simulink model "DSB_TC_Transmitter"  (R2022a)
settings: Solver=FixedStepDiscrete  StartTime=0.0  StopTime=inf  RelTol=1e-3
libraries: dspsnks4 x1, commanapbnd3 x1, dspvision x1, dspsigops x1, matrix_library x1
settings Model: Creator=vovan  LastModifiedBy=vovan

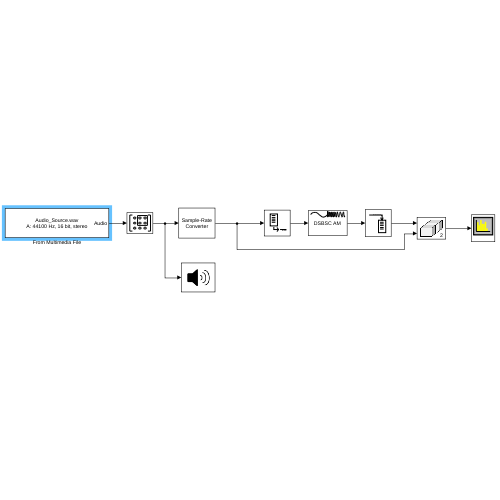
[thumbnail: Simulink's stored preview of the top-level diagram]
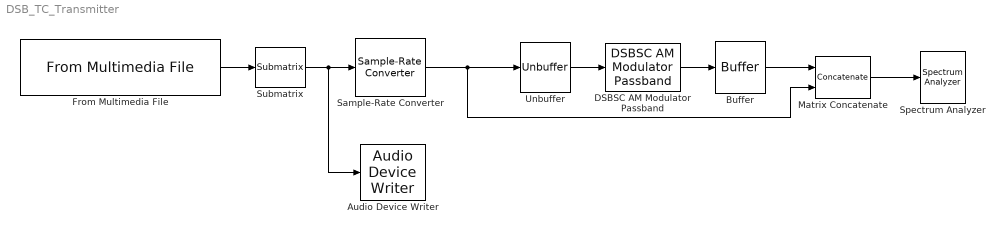
== system DSB_TC_Transmitter ==
  Audio Device Writer : dspsnks4/Audio Device Writer  Driver=ALSA  Device=Default  InheritSampleRate=on  SampleRate=44100  BitDepth=16-bit integer  BufferSize=4096  NumBuffers=10  DefaultOutputChannelMapping=on  OutputChannelMapping=1:2  OutputNumUnderrunSamples=off  DriverIdx=8  DeviceWarnFlag=''
  Buffer : Buffer  N=5000  OutputFrames=off
  DSBSC AM Modulator Passband : commanapbnd3/DSBSC AM Modulator Passband  Fc=60e3  Ph=0
      settings: SourceProductBaseCode=CM
  From Multimedia File : dspvision/From Multimedia File  inputFilename=./Audio_Source.wav  readRange=[1 Inf]  loop=on  numPlays=inf  outputStreams=Audio only  videoDataType=single  audioDataType=double  inheritSampleTime=on  userDefinedSampleTime=1/30  noAudioOutput=off  isIntensityVideo=off  fourcc=RGB  colorVideoFormat=Separate color signals  outputEOF=off  dataOrg=Column-major  audioFrameSize=1000  computeAudioFrameSize=off  outSamplingMode=Sample based
  Matrix Concatenate : Concatenate  Mode=Multidimensional array  ConcatenateDimension=2
  Sample-Rate Converter : dspsigops/Sample-Rate Converter  InputSampleRate=44100  OutputSampleRate=5*44100  OutputRateTolerance=0  Bandwidth=40e3  StopbandAttenuation=80  SimulateUsing=Code generation
      settings: SourceProductBaseCode=DS
  Spectrum Analyzer : SpectrumAnalyzer
  Submatrix : matrix_library/Submatrix  RowSpan=All rows  RowStartMode=First  RowStartIndex=1  RowEndMode=Last  RowEndIndex=1  ColSpan=Range of columns  ColStartMode=First  ColStartIndex=1  ColEndMode=Index  ColEndIndex=1
      settings: SourceProductBaseCode=SL
  Unbuffer : Unbuffer
  wires:
  From Multimedia File/1 -> Submatrix/1
  Sample-Rate Converter/1 -> Matrix Concatenate/2, Unbuffer/1
  DSBSC AM Modulator Passband/1 -> Buffer/1
  Unbuffer/1 -> DSBSC AM Modulator Passband/1
  Buffer/1 -> Matrix Concatenate/1
  Submatrix/1 -> Audio Device Writer/1, Sample-Rate Converter/1
  Matrix Concatenate/1 -> Spectrum Analyzer/1
